simulink model "MillingCircuit_openLoop"  (R2024a)
settings: Solver=ode23s  StartTime=0.0  StopTime=20  MaxStep=0.01  RelTol=1e-3
undefined symbols (not defined in the file): Q_mfo, Q_mso, Q_mwo
settings Model: Creator=tmlouw  LastModifiedBy=tmlouw

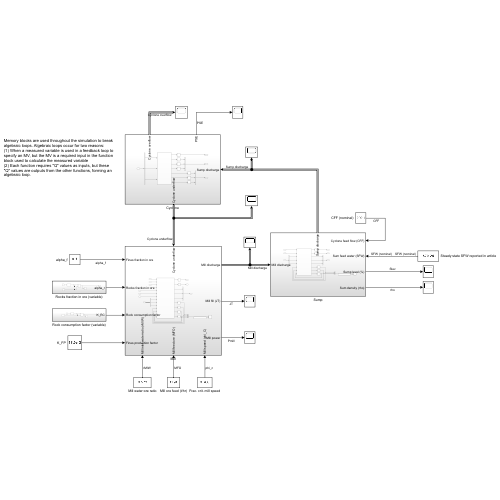
[thumbnail: Simulink's stored preview of the top-level diagram]
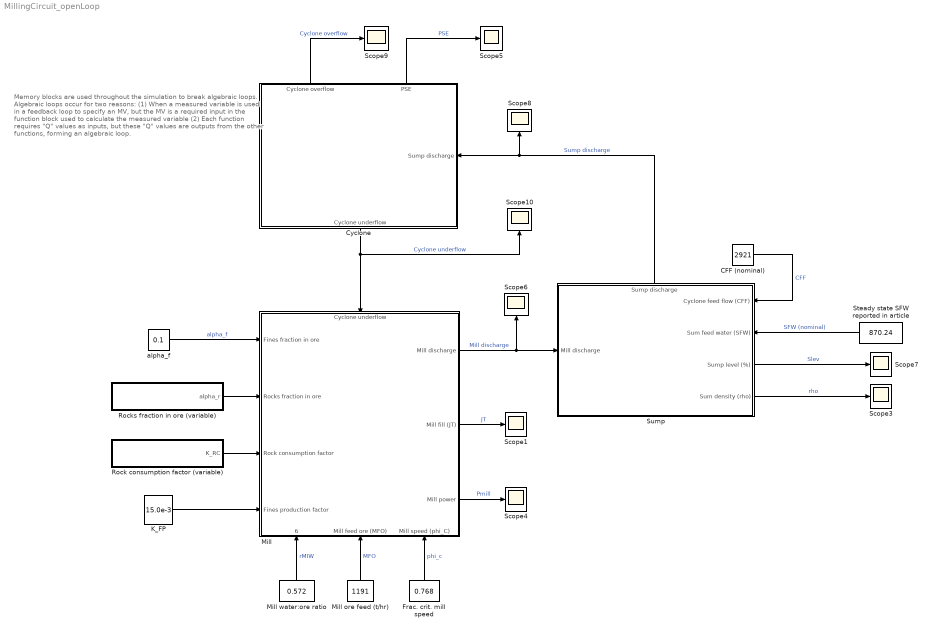
== system MillingCircuit_openLoop ==
  note: Memory blocks are used throughout the simulation to break algebraic loops. Algebraic loops occur for two reasons:
      | (1) When a measured variable is used in a feedback loop to specify an MV, but the MV is a required input in the function block used to calculate the measured variable
      | (2) Each function requires "Q" values as inputs, but these "Q" values are outputs from the other functions, forming an algebraic loop.
  CFF (nominal) : Constant  Value=2921
  Cyclone : Subsystem
      settings: PortSchema="{\"entries\":[{\"content\":{\"sides\":[{\"content\":{\"connectorIds\":[\"In1\"]},\"type\":\"ConnectorPlacement.EquallySpacedRectSide\",\"uuid\":\"e004a590-ab7d-4f12-a32b-87c0f3362931\"},{\"content\":{\"side\":\"RIGHT\"},\"type\":\"ConnectorPlacement.EquallySpacedRectSide\",\"uuid\":\"81f63357-3f4a-425b-a75c-7db5f55a4185\"},{\"content\":{\"connectorIds\":[\"Out2\",\"Out3\"],\"side\":\"TOP\"},\"type\":\"ConnectorPlacement.EquallySpacedRectSide\",\"uuid\":\"f49d5994-2e55-470a-b3f7-48bac8f55a82\"},{\"content\":{\"connectorIds\":[\"Out1\"],\"side\":\"BOTTOM\"},\"type\":\"ConnectorPlacement.EquallySpacedRectSide\",\"uuid\":\"f2576521-315b-4e2b-88a5-9b95980ef6dc\"}]},\"type\":\"ConnectorPlacement.EquallySpacedConnector\",\"uuid\":\"db23bcd0-405b-40f3-9326-1e4e7e72f851\"}],\"packageUris\":[\"http://schema.mathworks.com/mf0/Connector/R2020b\"],\"version\":\"1.0\"}"
  Frac. crit. mill speed : Constant  Value=0.768
  K_FP : Constant  Value=15.0e-3
  Mill : Subsystem
      settings: PortSchema="{\"entries\":[{\"content\":{\"sides\":[{\"content\":{\"connectorIds\":[\"In1\",\"In2\",\"In3\",\"In4\"]},\"type\":\"ConnectorPlacement.EquallySpacedRectSide\",\"uuid\":\"96805061-b1fe-4613-bdfe-c0403b68937d\"},{\"content\":{\"connectorIds\":[\"Out1\",\"Out2\",\"Out3\"],\"side\":\"RIGHT\"},\"type\":\"ConnectorPlacement.EquallySpacedRectSide\",\"uuid\":\"6c17841b-9594-4814-b3ce-f10677336251\"},{\"content\":{\"connectorIds\":[\"In5\"],\"side\":\"TOP\"},\"type\":\"ConnectorPlacement.EquallySpacedRectSide\",\"uuid\":\"6745fb07-3caa-4476-84a8-ded69789aedb\"},{\"content\":{\"connectorIds\":[\"In6\",\"In7\",\"In8\"],\"side\":\"BOTTOM\"},\"type\":\"ConnectorPlacement.EquallySpacedRectSide\",\"uuid\":\"985bb3c8-cd2a-4950-9ac1-ea614b478f36\"}]},\"type\":\"ConnectorPlacement.EquallySpacedConnector\",\"uuid\":\"041c7e0e-15c3-4fa4-bb53-6944ed039480\"}],\"packageUris\":[\"http://schema.mathworks.com/mf0/Connector/R2020b\"],\"version\":\"1.0\"}"
  Mill ore feed (t/hr) : Constant  Value=1191
  Mill water:ore ratio : Constant  Value=0.572
  Rock consumption factor (variable) : Subsystem
  Rocks fraction in ore (variable) : Subsystem
  Scope{1,3..10} (9 alike) : Scope
  Steady state SFW reported in article : Constant  Value=870.24
  Sump : Subsystem
      settings: PortSchema="{\"entries\":[{\"content\":{\"sides\":[{\"content\":{\"connectorIds\":[\"In1\"]},\"type\":\"ConnectorPlacement.EquallySpacedRectSide\",\"uuid\":\"4a068f6d-5fe1-4cb3-a916-3556d51fbafc\"},{\"content\":{\"connectorIds\":[\"In2\",\"In3\",\"Out1\",\"Out2\"],\"side\":\"RIGHT\"},\"type\":\"ConnectorPlacement.EquallySpacedRectSide\",\"uuid\":\"4fd936c1-8f9e-49fb-973c-89f6d774d731\"},{\"content\":{\"connectorIds\":[\"Out3\"],\"side\":\"TOP\"},\"type\":\"ConnectorPlacement.EquallySpacedRectSide\",\"uuid\":\"29d08788-fe4e-4f4a-9156-74b867964639\"}]},\"type\":\"ConnectorPlacement.EquallySpacedConnector\",\"uuid\":\"9bde5f39-013c-4aea-8ac6-be7cf98bab97\"}],\"packageUris\":[\"http://schema.mathworks.com/mf0/Connector/R2020b\"],\"version\":\"1.0\"}"
  alpha_f : Constant  Value=0.1
  wires:
  Cyclone/2(PSE) -> Scope5/1  "PSE"
  Sump/3(Sump discharge) -> Cyclone/1(Sump discharge), Scope8/1  "Sump discharge"
  Sump/2(Sum density (rho)) -> Scope3/1  "rho"
  Mill ore feed (t/hr)/1 -> Mill/7(Mill feed ore (MFO))  "MFO"
  Mill water:ore ratio/1 -> Mill/6(Mill inlet water ratio (rMIW))  "rMIW"
  Frac. crit. mill speed/1 -> Mill/8(Mill speed (phi_C))  "phi_c"
  Mill/3(Mill power) -> Scope4/1  "Pmill"
  Mill/2(Mill fill (JT)) -> Scope1/1  "JT"
  Mill/1(Mill discharge) -> Sump/1(Mill discharge), Scope6/1  "Mill discharge"
  Sump/1(Sump level (%)) -> Scope7/1  "Slev"
  CFF (nominal)/1 -> Sump/2(Cyclone feed flow (CFF))  "CFF"
  Steady state SFW reported in article/1 -> Sump/3(Sum feed water (SFW))  "SFW (nominal)"
  Cyclone/1(Cyclone underflow) -> Scope10/1, Mill/5(Cyclone underflow)  "Cyclone underflow"
  alpha_f/1 -> Mill/1(Fines fraction in ore)  "alpha_f"
  Cyclone/3(Cyclone overflow) -> Scope9/1  "Cyclone overflow"
  K_FP/1 -> Mill/4(Fines production factor)
  Rocks fraction in ore (variable)/1(alpha_r) -> Mill/2(Rocks fraction in ore)
  Rock consumption factor (variable)/1(K_RC) -> Mill/3(Rock consumption factor)

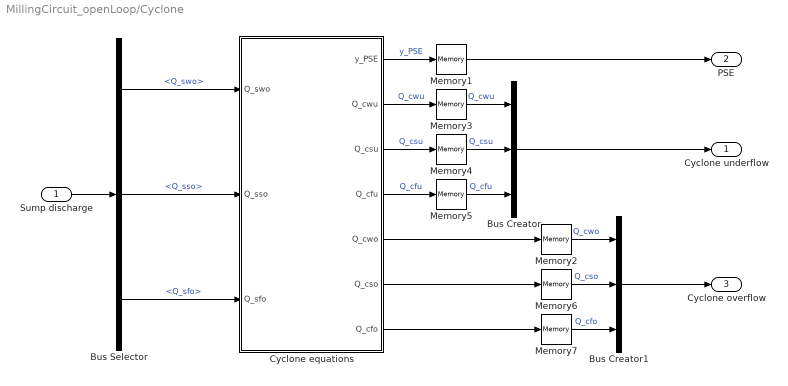
== system MillingCircuit_openLoop/Cyclone ==
  Sump discharge : Inport
  Bus Creator : BusCreator  Inputs=3
  Bus Creator1 : BusCreator  Inputs=3
  Bus Selector : BusSelector  OutputSignals=Q_swo,Q_sso,Q_sfo
  Cyclone equations : MATLAB Function  TreatAsAtomicUnit=on
  Memory1 : Memory  InitialCondition=37.9
  Memory2 : Memory  InitialCondition=1551.5
  Memory3 : Memory  InitialCondition=342.4747
  Memory4 : Memory  InitialCondition=654.4822
  Memory5 : Memory  InitialCondition=31.1095
  Memory6 : Memory  InitialCondition=372.2295
  Memory7 : Memory  InitialCondition=140.935
  Cyclone underflow : Outport
  PSE : Outport  Port=2
  Cyclone overflow : Outport  Port=3
  wires:
  Bus Selector/3 -> Cyclone equations/3(Q_sfo)  "<Q_sfo>"
  Cyclone equations/1(y_PSE) -> Memory1/1  "y_PSE"
  Bus Selector/2 -> Cyclone equations/2(Q_sso)  "<Q_sso>"
  Memory1/1 -> PSE/1
  Sump discharge/1 -> Bus Selector/1
  Bus Selector/1 -> Cyclone equations/1(Q_swo)  "<Q_swo>"
  Cyclone equations/4(Q_cfu) -> Memory5/1  "Q_cfu"
  Cyclone equations/3(Q_csu) -> Memory4/1  "Q_csu"
  Cyclone equations/2(Q_cwu) -> Memory3/1  "Q_cwu"
  Bus Creator/1 -> Cyclone underflow/1
  Memory3/1 -> Bus Creator/1  "Q_cwu"
  Memory4/1 -> Bus Creator/2  "Q_csu"
  Memory5/1 -> Bus Creator/3  "Q_cfu"
  Memory7/1 -> Bus Creator1/3  "Q_cfo"
  Memory2/1 -> Bus Creator1/1  "Q_cwo"
  Bus Creator1/1 -> Cyclone overflow/1
  Memory6/1 -> Bus Creator1/2  "Q_cso"
  Cyclone equations/5(Q_cwo) -> Memory2/1
  Cyclone equations/6(Q_cso) -> Memory6/1
  Cyclone equations/7(Q_cfo) -> Memory7/1

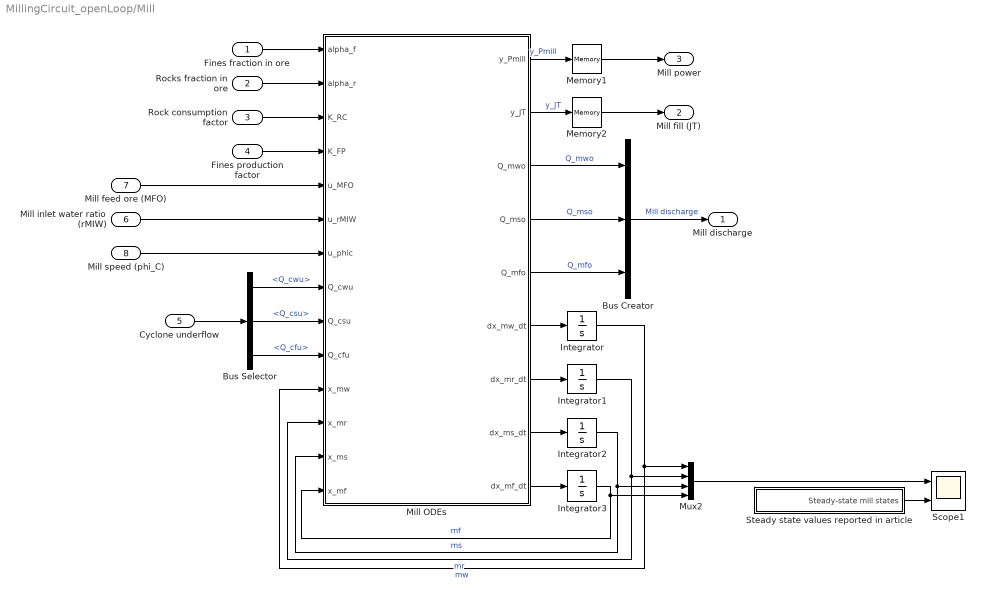
== system MillingCircuit_openLoop/Mill ==
  Fines fraction in ore : Inport
  Rocks fraction in ore : Inport  Port=2
  Rock consumption factor : Inport  Port=3
  Fines production factor : Inport  Port=4
  Cyclone underflow : Inport  Port=5
  Mill inlet water ratio (rMIW) : Inport  Port=6
  Mill feed ore (MFO) : Inport  Port=7
  Mill speed (phi_C) : Inport  Port=8
  Bus Creator : BusCreator  Inputs=Q_mwo,Q_mso,Q_mfo
  Bus Selector : BusSelector  OutputSignals=Q_cwu,Q_csu,Q_cfu
  Integrator : Integrator  InitialCondition=31.4051  LimitOutput=on  LowerSaturationLimit=0
  Integrator1 : Integrator  InitialCondition=9.8378  LimitOutput=on  LowerSaturationLimit=0
  Integrator2 : Integrator  InitialCondition=31.1314  LimitOutput=on  LowerSaturationLimit=0
  Integrator3 : Integrator  InitialCondition=5.2166  LimitOutput=on  LowerSaturationLimit=0
  Memory1 : Memory  InitialCondition=14.812
  Memory2 : Memory  InitialCondition=0.328
  Mill ODEs : MATLAB Function  TreatAsAtomicUnit=on
  Mux2 : Mux
  Scope1 : Scope  NumInputPorts=2
  Steady state values reported in article : Subsystem
  Mill discharge : Outport
  Mill fill (JT) : Outport  Port=2
  Mill power : Outport  Port=3
  wires:
  Mill ODEs/8(dx_ms_dt) -> Integrator2/1
  Mill ODEs/6(dx_mw_dt) -> Integrator/1
  Integrator3/1 -> Mill ODEs/14(x_mf), Mux2/4  "mf"
  Mill ODEs/7(dx_mr_dt) -> Integrator1/1
  Mill feed ore (MFO)/1 -> Mill ODEs/5(u_MFO)
  Mill ODEs/9(dx_mf_dt) -> Integrator3/1
  Mill speed (phi_C)/1 -> Mill ODEs/7(u_phic)
  Mill ODEs/2(y_JT) -> Memory2/1  "y_JT"
  Mill inlet water ratio (rMIW)/1 -> Mill ODEs/6(u_rMIW)
  Mill ODEs/3(Q_mwo) -> Bus Creator/1  "Q_mwo"
  Mill ODEs/5(Q_mfo) -> Bus Creator/3  "Q_mfo"
  Mill ODEs/4(Q_mso) -> Bus Creator/2  "Q_mso"
  Mill ODEs/1(y_Pmill) -> Memory1/1  "y_Pmill"
  Mux2/1 -> Scope1/1
  Integrator/1 -> Mill ODEs/11(x_mw), Mux2/1  "mw"
  Integrator2/1 -> Mill ODEs/13(x_ms), Mux2/3  "ms"
  Integrator1/1 -> Mill ODEs/12(x_mr), Mux2/2  "mr"
  Memory1/1 -> Mill power/1
  Memory2/1 -> Mill fill (JT)/1
  Fines fraction in ore/1 -> Mill ODEs/1(alpha_f)
  Rocks fraction in ore/1 -> Mill ODEs/2(alpha_r)
  Rock consumption factor/1 -> Mill ODEs/3(K_RC)
  Fines production factor/1 -> Mill ODEs/4(K_FP)
  Bus Creator/1 -> Mill discharge/1  "Mill discharge"
  Cyclone underflow/1 -> Bus Selector/1
  Bus Selector/1 -> Mill ODEs/8(Q_cwu)  "<Q_cwu>"
  Bus Selector/2 -> Mill ODEs/9(Q_csu)  "<Q_csu>"
  Bus Selector/3 -> Mill ODEs/10(Q_cfu)  "<Q_cfu>"
  Steady state values reported in article/1(Steady-state mill states) -> Scope1/2

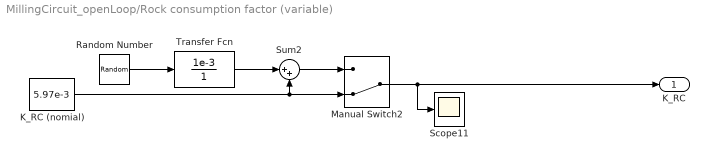
== system MillingCircuit_openLoop/Rock consumption factor (variable) ==
  K_RC (nomial) : Constant  Value=5.97e-3
  Manual Switch2 : ManualSwitch  CurrentSetting=0
  Random Number : RandomNumber  SampleTime=4
  Scope11 : Scope
  Sum2 : Sum  Inputs=|++
  Transfer Fcn : TransferFcn  Numerator=[1e-3]  Denominator=[0 1]
  K_RC : Outport
  wires:
  Manual Switch2/1 -> K_RC/1, Scope11/1
  Transfer Fcn/1 -> Sum2/1
  K_RC (nomial)/1 -> Manual Switch2/2, Sum2/2
  Random Number/1 -> Transfer Fcn/1
  Sum2/1 -> Manual Switch2/1

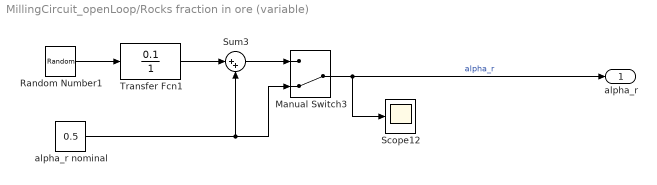
== system MillingCircuit_openLoop/Rocks fraction in ore (variable) ==
  Manual Switch3 : ManualSwitch  CurrentSetting=0
  Random Number1 : RandomNumber  SampleTime=2
  Scope12 : Scope
  Sum3 : Sum  Inputs=|++
  Transfer Fcn1 : TransferFcn  Numerator=[0.1]  Denominator=[0 1]
  alpha_r nominal : Constant  Value=0.5
  alpha_r : Outport
  wires:
  Random Number1/1 -> Transfer Fcn1/1
  Manual Switch3/1 -> alpha_r/1, Scope12/1  "alpha_r"
  alpha_r nominal/1 -> Manual Switch3/2, Sum3/2
  Sum3/1 -> Manual Switch3/1
  Transfer Fcn1/1 -> Sum3/1

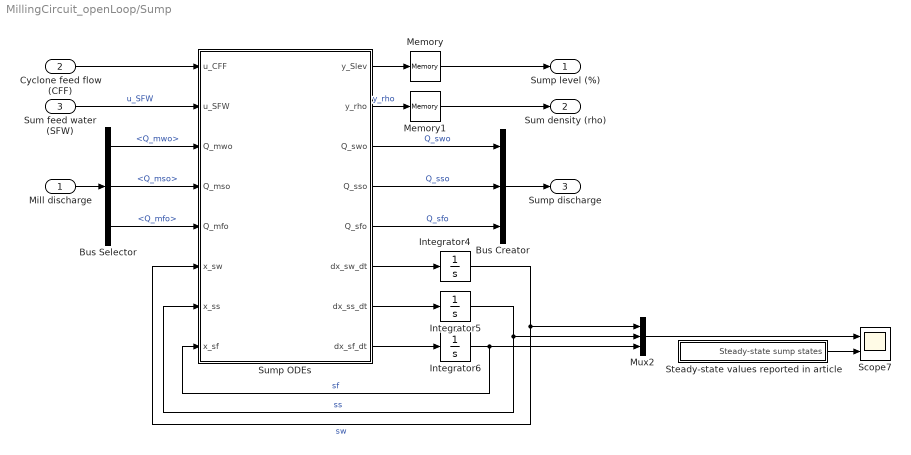
== system MillingCircuit_openLoop/Sump ==
  Mill discharge : Inport
  Cyclone feed flow (CFF) : Inport  Port=2
  Sum feed water (SFW) : Inport  Port=3
  Bus Creator : BusCreator  Inputs=3
  Bus Selector : BusSelector  OutputSignals=Q_mwo,Q_mso,Q_mfo
  Integrator4 : Integrator  InitialCondition=133.187  LimitOutput=on  LowerSaturationLimit=0
  Integrator5 : Integrator  InitialCondition=72.1996  LimitOutput=on  LowerSaturationLimit=1e-3
  Integrator6 : Integrator  InitialCondition=12.09  LimitOutput=on  LowerSaturationLimit=0
  Memory : Memory  InitialCondition=59.4
  Memory1 : Memory  InitialCondition=1.7733
  Mux2 : Mux  Inputs=3
  Scope7 : Scope  NumInputPorts=2
  Steady-state values reported in article : Subsystem
  Sump ODEs : MATLAB Function  TreatAsAtomicUnit=on
  Sump level (%) : Outport
  Sum density (rho) : Outport  Port=2
  Sump discharge : Outport  Port=3
  wires:
  Integrator4/1 -> Sump ODEs/6(x_sw), Mux2/1  "sw"
  Sum feed water (SFW)/1 -> Sump ODEs/2(u_SFW)  "u_SFW"
  Sump ODEs/4(Q_sso) -> Bus Creator/2  "Q_sso"
  Sump ODEs/6(dx_sw_dt) -> Integrator4/1
  Sump ODEs/7(dx_ss_dt) -> Integrator5/1
  Bus Selector/3 -> Sump ODEs/5(Q_mfo)  "<Q_mfo>"
  Sump ODEs/8(dx_sf_dt) -> Integrator6/1
  Integrator6/1 -> Mux2/3, Sump ODEs/8(x_sf)  "sf"
  Integrator5/1 -> Sump ODEs/7(x_ss), Mux2/2  "ss"
  Cyclone feed flow (CFF)/1 -> Sump ODEs/1(u_CFF)
  Sump ODEs/2(y_rho) -> Memory1/1  "y_rho"
  Sump ODEs/3(Q_swo) -> Bus Creator/1  "Q_swo"
  Sump ODEs/5(Q_sfo) -> Bus Creator/3  "Q_sfo"
  Sump ODEs/1(y_Slev) -> Memory/1
  Memory/1 -> Sump level (%)/1
  Memory1/1 -> Sum density (rho)/1
  Mux2/1 -> Scope7/1
  Mill discharge/1 -> Bus Selector/1
  Bus Creator/1 -> Sump discharge/1
  Bus Selector/2 -> Sump ODEs/4(Q_mso)  "<Q_mso>"
  Bus Selector/1 -> Sump ODEs/3(Q_mwo)  "<Q_mwo>"
  Steady-state values reported in article/1(Steady-state sump states) -> Scope7/2

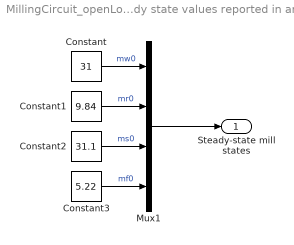
== system MillingCircuit_openLoop/Mill/Steady state values reported in article ==
  Constant : Constant  Value=31
  Constant1 : Constant  Value=9.84
  Constant2 : Constant  Value=31.1
  Constant3 : Constant  Value=5.22
  Mux1 : Mux
  Steady-state mill states : Outport
  wires:
  Constant1/1 -> Mux1/2  "mr0"
  Constant3/1 -> Mux1/4  "mf0"
  Constant/1 -> Mux1/1  "mw0"
  Mux1/1 -> Steady-state mill states/1
  Constant2/1 -> Mux1/3  "ms0"

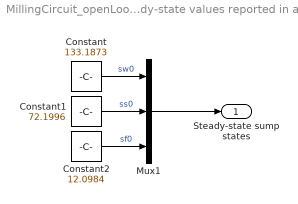
== system MillingCircuit_openLoop/Sump/Steady-state values reported in article ==
  Constant : Constant  Value=133.1873
  Constant1 : Constant  Value=72.1996
  Constant2 : Constant  Value=12.0984
  Mux1 : Mux  Inputs=3
  Steady-state sump states : Outport
  wires:
  Constant1/1 -> Mux1/2  "ss0"
  Constant/1 -> Mux1/1  "sw0"
  Mux1/1 -> Steady-state sump states/1
  Constant2/1 -> Mux1/3  "sf0"

== matlab function MillingCircuit_openLoop/Sump/Sump ODEs ==
  data: y_Slev output; u_CFF input; y_rho output; Q_swo output; Q_sso output; Q_sfo output; u_SFW input; dx_sw_dt output; Q_mwo input; Q_mso input; Q_mfo input; x_sw input; x_ss input; x_sf input; dx_ss_dt output; dx_sf_dt output
function [y_Slev, y_rho, Q_swo, Q_sso, Q_sfo, dx_sw_dt, dx_ss_dt, dx_sf_dt] = SumpModel(u_CFF, u_SFW, Q_mwo, Q_mso, Q_mfo, x_sw, x_ss, x_sf)
% Inputs:
%  u_SFW:  (m3/h), sump feed water flowrate
%  u_CFF:  (m3/h), cyclone feed flowrate

% Shared parameters
rho_o = 3.2;  % t/m3, density of ore
rho_w = 1.0;  % t/m3, density of water

% Sump parameters
v_sump = 345.8; % m3, sump volume

% Sump discharge flowrates
Q_swo = u_CFF*( x_sw / (x_ss + x_sw) ); % m3/hr, sump water discharge flowrate
Q_sso = u_CFF*( x_ss / (x_ss + x_sw) ); % m3/hr, sump solids discharge flowrate
Q_sfo = u_CFF*( x_sf / (x_ss + x_sw) ); % m3/hr, sump fines discharge flowrate

% Measured variables
y_Slev = 100*(x_ss + x_sw)/v_sump;  % (%), sump level
y_rho = ( rho_w*Q_swo + rho_o*Q_sso ) / ( Q_swo + Q_sso ); % t/m3, sump discharge density

% Accum. = in    - out   + feed water
dx_sw_dt = Q_mwo - Q_swo + u_SFW;  % x_sw (m3), volume of water in sump
dx_ss_dt = Q_mso - Q_sso;          % x_ss (m3), volume of solids in sump
dx_sf_dt = Q_mfo - Q_sfo;          % x_sf (m3), volume of fines in sump

== matlab function MillingCircuit_openLoop/Mill/Mill ODEs ==
  data: alpha_f input; alpha_r input; K_RC input; K_FP input; y_Pmill output; y_JT output; Q_mwo output; Q_mso output; Q_mfo output; u_MFO input; dx_mw_dt output; dx_mr_dt output; dx_ms_dt output; dx_mf_dt output; u_rMIW input; u_phic input; Q_cwu input; Q_csu input; Q_cfu input; x_mw input; x_mr input; x_ms input; x_mf input
function [y_Pmill, y_JT, Q_mwo, Q_mso, Q_mfo, dx_mw_dt, dx_mr_dt, dx_ms_dt, dx_mf_dt] = MillModel(alpha_f, alpha_r, K_RC, K_FP, u_MFO, u_rMIW, u_phic, Q_cwu, Q_csu, Q_cfu, x_mw, x_mr, x_ms, x_mf)
% Inputs:
%  u_MFO:  (t/h), mill feed ore
%  u_rMIW: (~), ratio of mill inlet water to feed ore
%  u_phic: (~), fraction of critical mill speed

% Shared parameters
rho_o = 3.2;  % t/m3, density of ore
rho_w = 1.0;  % t/m3, density of water

% Ore properties (potential disturbances)
% alpha_f = 0.1; % ~, mass fraction of fines in the feed ore
% alpha_r = 0.5; % ~, mass fraction of rocks in the feed ore
% K_RC = 5.97e-3; % MWh/t, rock consumption factor
% K_FP = 15.0e-3; % MWh/t, fines production factor

% Mill parameters
delta_s = 0.0911; % ~, power parameter for fraction solids in mill
delta_v = 0.0911; % ~, power parameter for volume of mill filled
phi_N = 0.7;      % ~, rheology normalisation factor
J_TPmax = 0.23;   % ~, fraction of mill filled at max power draw

d_q = 114.7; % 1/hr, discharge rate
eps_0 = 0.6; % ~, max fraction of solids at zero slurry flow

K_FPJT = 20;    % ~, fractional change in fines production factor / fractional mill filling
P_max = 19.685;   % MW, max mill power draw 

v_mill = 540.9; % m3, mill volume
x_mb = 105.41; % m3, volume of balls in mill

% Note that "solids" includes fines and coarse, thus: 
%   alpha_f < alpha_s = 1-alpha_r
%   x_ms > m_mf

% Intermediate variables
% The model sets phi = 0 if 1 - (1/eps_0 - 1)*x_ms/x_mw  ) < 0
phi = sqrt(  max(0, 1 - (eps_0^-1 - 1)*x_ms/x_mw  ) ); % ~, rheology factor

% Measured variables
y_JT = ( x_mw + x_ms + x_mr + x_mb ) / v_mill;  % m3, fraction of mill filled
y_Pmill = P_max*u_phic*( 1 - delta_v*(y_JT/J_TPmax - 1)^2 - delta_s*(phi/phi_N - 1)^2 );  % MW, mill power draw

% Mill feed flowrates
Q_mwf = u_rMIW*u_MFO/rho_w;         % m3/hr, mill water feed flowrate
Q_mrf = alpha_r*u_MFO/rho_o;        % m3/hr, mill rock feed flowrate
Q_msf = (1 - alpha_r)*u_MFO/rho_o;  % m3/hr, mill ore feed flowrate
Q_mff = alpha_f*u_MFO/rho_o;        % m3/hr, mill fines feed flowrate

% Mill discharge flowrates
Q_mwo = (phi*d_q*x_mw) * ( x_mw / (x_ms + x_mw) ); % m3/hr, mill water discharge flowrate
Q_mso = (phi*d_q*x_mw) * ( x_ms / (x_ms + x_mw) ); % m3/hr, mill solids discharge flowrate
Q_mfo = (phi*d_q*x_mw) * ( x_mf / (x_ms + x_mw) ); % m3/hr, mill fines discharge flowrate

% Consumption and production
Q_RC = y_Pmill/(rho_o*K_RC) * ( x_mr/(x_mr + x_ms) );       % m3/hr, rock consumption
Q_FP = y_Pmill/(rho_o*K_FP) / ( 1 + K_FPJT*(y_JT - J_TPmax) ); % m3/hr, fines production

% Accum. = in    - out   + cyclone + rock consumption + fines production
dx_mw_dt = Q_mwf - Q_mwo + Q_cwu;                   % x_mw (m3), volume of water in mill
dx_mr_dt = Q_mrf                   - Q_RC;          % x_mr (m3), volume of rocks in mill, too large to discharge
dx_ms_dt = Q_msf - Q_mso + Q_csu   + Q_RC;          % x_ms (m3), volume of solids in mill
dx_mf_dt = Q_mff - Q_mfo + Q_cfu          + Q_FP;   % x_mf (m3), volume of fines in mill

== matlab function MillingCircuit_openLoop/Cyclone/Cyclone equations ==
  data: y_PSE output; Q_swo input; Q_sso input; Q_sfo input; Q_cwu output; Q_csu output; Q_cfu output; Q_cwo output; Q_cso output; Q_cfo output
function [y_PSE, Q_cwu, Q_csu, Q_cfu, Q_cwo, Q_cso, Q_cfo] = CycloneModel(Q_swo, Q_sso, Q_sfo)
% Inputs:
%  u_SFW:  (m3/h), sump feed water flowrate
%  u_CFF:  (m3/h), cyclone feed flowrate

% Cyclone parameters
C1 = 0.7; % ~
C2 = 0.7; % ~
C3 = 4;   % ~
alpha_su = 0.1185; % ~
eps_C = 2528; % m3/h

% Intermediate variables
u_CFF = Q_swo + Q_sso;
Fi = Q_sso/u_CFF;   % ~, fraction solids in the cyclone feed
Q_ccu = (Q_sso - Q_sfo)*(  1 - C1*exp(-u_CFF/eps_C)  ) ...
                       *(  1 - ( Fi/C2 )^C3  ) ...
                       *(  1 - ( Q_sfo/Q_sso )^C3 );     % m3/hr, cyclone coarse underflow flowrate

Fu = C2 - (C2 - Fi)*exp( -Q_ccu/(alpha_su*eps_C) );  % ~ fraction solids in the underflow

% Cyclone underflow flowrates
Q_cwu = Q_swo * (1 - Fu)*Q_ccu / (Fu*Q_swo + Fu*Q_sfo - Q_sfo + 1e-9);  % m3/hr, cyclone water underflow flowrate
Q_cfu = Q_sfo * (1 - Fu)*Q_ccu / (Fu*Q_swo + Fu*Q_sfo - Q_sfo + 1e-9);  % m3/hr, cyclone fines underflow flowrate 
Q_csu = Q_ccu + Q_cfu;  % m3/hr, cyclone solids underflow flowrate

% Cyclone overflow flowrates
Q_cwo = Q_swo - Q_cwu;
Q_cso = Q_sso - Q_csu;
Q_cfo = Q_sfo - Q_cfu;


% Measured variables
y_PSE = 100*Q_cfo/Q_cso;
